simulink model "point_system"  (R2016b)
settings: Solver=VariableStepAuto  StartTime=0.0  StopTime=10.0  RelTol=1e-3
settings Model: Creator=kevin  LastModifiedBy=kevin

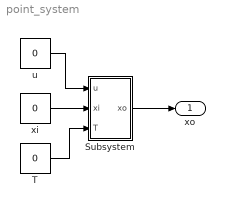
== system point_system ==
  Subsystem : Subsystem
  T : Constant  Value=0
  u : Constant  Value=0
  xi : Constant  Value=0
  xo : Outport
  wires:
  u/1 -> Subsystem/1(u)
  xi/1 -> Subsystem/2(xi)
  T/1 -> Subsystem/3(T)
  Subsystem/1(xo) -> xo/1

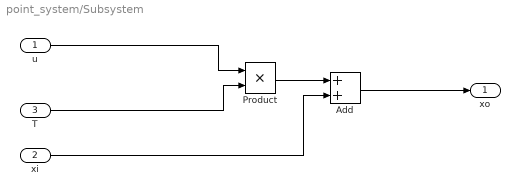
== system point_system/Subsystem ==
  u : Inport
  xi : Inport  Port=2
  T : Inport  Port=3
  Add : Sum
  Product : Product
  xo : Outport
  wires:
  Product/1 -> Add/1
  u/1 -> Product/1
  T/1 -> Product/2
  xi/1 -> Add/2
  Add/1 -> xo/1
